simulink model "dvb_s2_channel_2"  (R2025b)
settings: Solver=VariableStepAuto  StartTime=0.0  StopTime=1  RelTol=1e-3
undefined symbols (not defined in the file): GenBCHPoly, SNR
libraries: commsync2 x2, commfilt2 x2, commblkcod2 x2, commchan3 x1, commrflib2 x1, commdigbbndpm3 x1, simulink x1, dspsigops x1, commsink2 x1
settings Model: Creator=Пётр  LastModifiedBy=Пётр

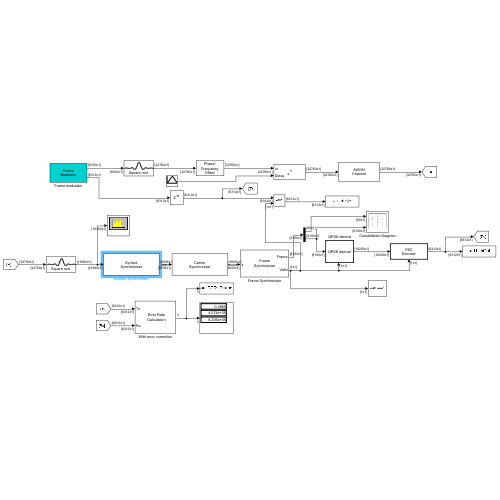
[thumbnail: Simulink's stored preview of the top-level diagram]
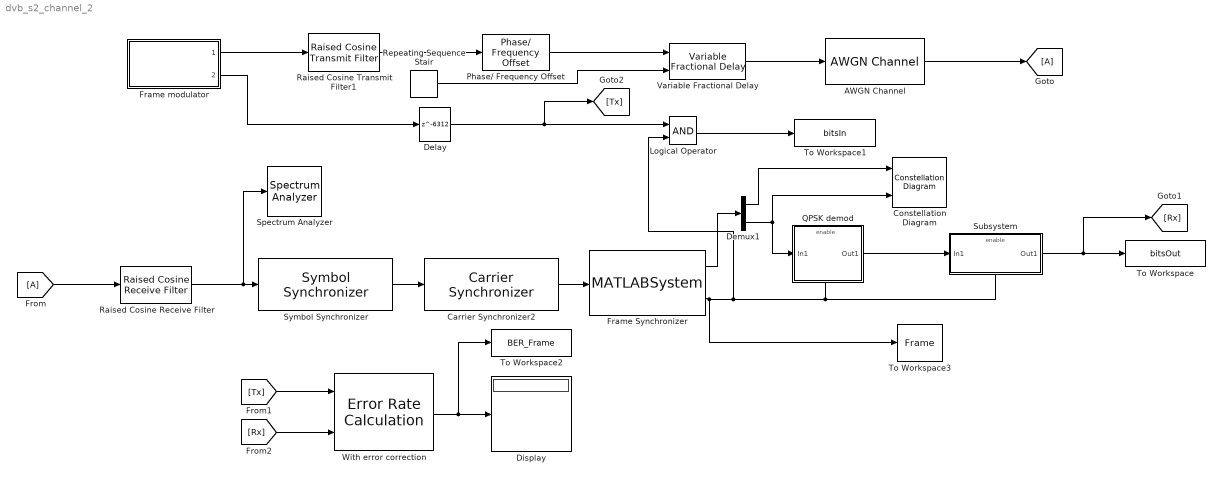
== system dvb_s2_channel_2 ==
  AWGN Channel : commchan3/AWGN Channel  LegacyMode=off  NoiseMethod="Signal to noise ratio  (SNR)"  noiseMode="Signal to noise ratio  (SNR)"  EbNo=10  EsNo=10  SNR=SNR  BitsPerSymbol=1  SignalPower=1  SpecifySymbolPeriod=off  SamplesPerSymbol=1  SymbolPeriod=1  VarianceSource=Parameter  Variance=1  RandomStream=Global stream  Seed=67  SimulateUsing=Code generation
  Carrier Synchronizer2 : commsync2/Carrier Synchronizer  Modulation=QPSK  ModulationPhaseOffset=Auto  CustomPhaseOffset=pi/2  SamplesPerSymbol=2  DampingFactor=0.707  NormalizedLoopBandwidth=0.01  EstimatedPhaseErrorOutputPort=off  SimulateUsing=Code generation
  Constellation Diagram : ConstellationDiagram  NumInputPorts=2  WindowPosition=[676.000000,240.000000,602.000000,517.000000,]  Visible=on  ScopeFrameLocation=window  SymbolsToDisplaySource=Property  SymbolsToDisplay=1000  ReferenceConstellation="[0.70711+0.70711i        -0.70711+0.70711i        -0.70711-0.70711i         0.70711-0.70711i]"  ShowLegend=on  MeasurementInterval=1000
  Delay : Delay  DelayLength=6312  InputProcessing=Columns as channels (frame based)  UseCircularBuffer=on
  Demux1 : Demux  Outputs=[90 8100]
  Display : Display
  Frame Synchronizer : MATLABSystem  System=FrameSynchronizer  Preamble=SOF  Threshold=14  OutputLength=8190  SimulateUsing=Interpreted execution
      mask Type: FrameSynchronizer
  Frame modulator : Subsystem  ReferencedSubsystem=FrameGenerator
  From : From
  Goto : Goto
  Logical Operator : Logic  AllPortsSameDT=off  OutDataTypeStr=boolean
  Phase/ Frequency Offset : commrflib2/Phase// Frequency Offset  phaseOffset=0  freqPort=off  freqOffset=1000
  QPSK demod : Subsystem
      mask Display: disp('QPSK demod')
  Raised Cosine Receive Filter : commfilt2/Raised Cosine Receive Filter  filtType=Square root  R=0.25  filtSpan=10  N=4  downFactor=2  downOffset=0  filterGain=1  InputProcessing=Columns as channels (frame based)  RateOptions=Enforce single-rate processing  framing=Mute  checkCoeff=off  variableName=rcRxFilt  currentFiltSpan=10  D=5  inputOffset=0  sampMode=Mute  saveAsFlag=0  rateMode=Downsampling  checkGain=Normalized  launchFVT=on  roundingMode=Floor  overflowMode=off  coeffDataTypeStr=Inherit: Same word length as input  coeffMin=[]  coeffMax=[]  coeffLastDataTypeStr=Inherit: Same word length as input  accumDataTypeStr=Inherit: Same as product output  accumLastDataTypeStr=Inherit: Same as product output  outputDataTypeStr=Inherit: Same as accumulator  outputMin=[]  outputMax=[]  outputLastDataTypeStr=Inherit: Same as accumulator
  Raised Cosine Transmit Filter1 : commfilt2/Raised Cosine Transmit Filter  filtType=Square root  R=0.2  filtSpan=10  N=4  filterGain=1  InputProcessing=Columns as channels (frame based)  RateOptions=Enforce single-rate processing  framing=Mute  checkCoeff=off  variableName=rcTxFilt1  checkGain=Normalized  sampMode=Mute  saveAsFlag=0  currentFiltSpan=10  D=(10)/2  launchFVT=on  roundingMode=Floor  overflowMode=off  coeffDataTypeStr=Inherit: Same word length as input  coeffMin=[]  coeffMax=[]  coeffLastDataTypeStr=Inherit: Same word length as input  outputDataTypeStr=Inherit: Same as accumulator  outputMin=[]  outputMax=[]  outputLastDataTypeStr=Inherit: Same as accumulator
  Repeating Sequence Stair : simulink/Sources/Repeating Sequence Stair  OutValues=[0:0.1:0.9 0.8:-0.1:0.1]  tsamp=-1  OutMin=[]  OutMax=[]  OutDataTypeStr=double  OutputDataTypeScalingMode=double  OutDataType=fixdt(0,8)  ConRadixGroup=Best Precision: Vector-wise  OutScaling=2^-12
  Spectrum Analyzer : SpectrumAnalyzer  WindowPosition=[42.000000,231.000000,567.000000,504.000000,]  Visible=on  ScopeFrameLocation=window  SampleRate=100000000  Span=1000000  StartFrequency=-500000  StopFrequency=500000  AveragingMethod=Exponential  YLimits=[-80.4688 19.4697]  ShowLegend=on  AllowFFTLengthLessThanSamplesPerUpdate=on
  Subsystem : Subsystem
      mask Display: disp('FEC\nDecoder')
  Symbol Synchronizer : commsync2/Symbol Synchronizer  Modulation=PAM/PSK/QAM  TimingErrorDetector=Gardner (non-data-aided)  SamplesPerSymbol=2  DampingFactor=1  NormalizedLoopBandwidth=0.01  DetectorGain=2.7  TimingErrorOutputPort=off  SimulateUsing=Code generation
  To Workspace : ToWorkspace  VariableName=bitsOut  SampleTime=-1
      settings: Save2DSignal=2-D array (concatenate along first dimension)
  To Workspace1 : ToWorkspace  VariableName=bitsIn  SampleTime=-1
      settings: Save2DSignal=2-D array (concatenate along first dimension)
  To Workspace2 : ToWorkspace  VariableName=BER_Frame  SampleTime=-1
      settings: Save2DSignal=2-D array (concatenate along first dimension)
  To Workspace3 : ToWorkspace  VariableName=Frame  SampleTime=-1
      settings: Save2DSignal=2-D array (concatenate along first dimension)
  Variable Fractional Delay : dspsigops/Variable Fractional Delay  mode=OBSOLETE  modeActive=Linear  L=4  FarrowL=4  R=10  alpha=1  dmax=400  InputProcessing=Columns as channels (frame based)  ic=0  noDFT=off  fallbackFIR=Clip to the minimum value necessary for centered kernel  fallbackFarrow=Clip to the minimum value necessary for centered kernel  roundingMode=Zero  overflowMode=off
  With error correction : commsink2/Error Rate Calculation  N=0  st_delay=0  cp_mode=Entire frame  subframe=[]  PMode=Port  WsName=ErrorVec  RsMode2=off  stop=off  numErr=100  maxBits=1e6
  wires:
  Frame modulator/1 -> Raised Cosine Transmit Filter1/1
  Repeating Sequence Stair/1 -> Variable Fractional Delay/2
  Raised Cosine Transmit Filter1/1 -> Phase/ Frequency Offset/1
  Variable Fractional Delay/1 -> AWGN Channel/1
  Frame Synchronizer/2 -> Logical Operator/2, Subsystem/Enable, QPSK demod/Enable, To Workspace3/1
  Phase/ Frequency Offset/1 -> Variable Fractional Delay/1
  Frame modulator/2 -> Delay/1
  QPSK demod/1(Out1) -> Subsystem/1(In1)
  Frame Synchronizer/1 -> Demux1/1
  Demux1/2 -> QPSK demod/1(In1), Constellation Diagram/2
  Demux1/1 -> Constellation Diagram/1
  Symbol Synchronizer/1 -> Carrier Synchronizer2/1
  AWGN Channel/1 -> Goto/1
  From/1 -> Raised Cosine Receive Filter/1
  Delay/1 -> [Tx], Logical Operator/1
  Logical Operator/1 -> To Workspace1/1
  With error correction/1 -> To Workspace2/1, Display/1
  [Tx] -> With error correction/1
  [Rx] -> With error correction/2
  Subsystem/1(Out1) -> [Rx], To Workspace/1
  Carrier Synchronizer2/1 -> Frame Synchronizer/1
  Raised Cosine Receive Filter/1 -> Symbol Synchronizer/1, Spectrum Analyzer/1

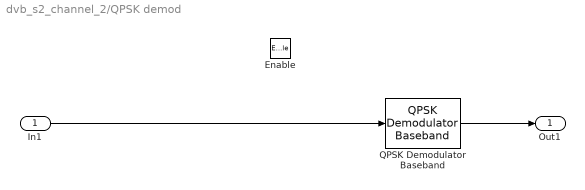
== system dvb_s2_channel_2/QPSK demod ==
  In1 : Inport
  Enable : EnablePort  StatesWhenEnabling=reset
  QPSK Demodulator Baseband : commdigbbndpm3/QPSK Demodulator Baseband  OutType=Bit  DecType=Approximate log-likelihood ratio  VarSource=Dialog  Variance=SNR  Dec=Binary  Ph=pi/4  outDtype1=Inherit via internal rule  outDtype2=Inherit via internal rule  derotateFactorWordLen=16  derotateFactorDataTypeStr=Inherit: Same word length as input  derotateFactorLastDataTypeStr=Inherit: Same word length as input
      settings: LibrarySourceBlock=|
      | commhdldigbbndpm/QPSK
      | Demodulator
      | Baseband
  Out1 : Outport
  wires:
  In1/1 -> QPSK Demodulator Baseband/1
  QPSK Demodulator Baseband/1 -> Out1/1

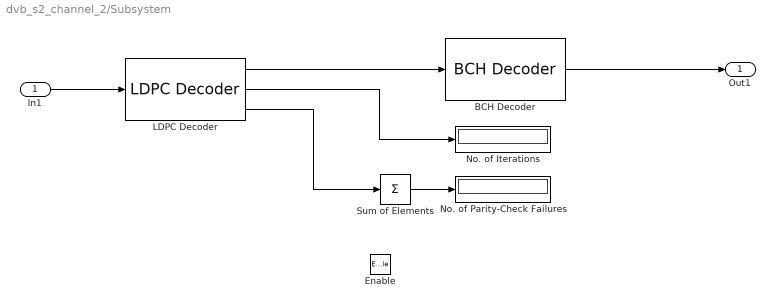
== system dvb_s2_channel_2/Subsystem ==
  In1 : Inport
  Enable : EnablePort
  BCH Decoder : commblkcod2/BCH Decoder  n=16383  k=16215  specShortening=on  shortenedK=6312  specGenPoly=on  genPoly=GenBCHPoly(12)  specPrimPoly=off  prPoly='X^4 + X + 1'  specDisableGenCheck=on  specPuncture=off  punctVec=[ones(8,1); zeros(2,1)]  specErasurePort=off  showNumErr=off
  LDPC Decoder : commblkcod2/LDPC Decoder  ParityCheckMat=LDPC25Matrix  OutputFmt=Information part  DecisionType=Hard decision  OutputDataType=boolean  NumIter=50  DoParityCheck=off  OutputNumIter=on  OutputFinalChecks=on
  No. of Iterations : Display
  No. of Parity-Check Failures : Display
  Sum of Elements : Sum  Inputs=+
  Out1 : Outport
  wires:
  BCH Decoder/1 -> Out1/1
  Sum of Elements/1 -> No. of Parity-Check Failures/1
  In1/1 -> LDPC Decoder/1
  LDPC Decoder/1 -> BCH Decoder/1
  LDPC Decoder/3 -> Sum of Elements/1
  LDPC Decoder/2 -> No. of Iterations/1
